simulink model "SSSTSMCC_SIM2augr"  (R2021a)
settings: Solver=ode23  StartTime=0.0  StopTime=T_s  RelTol=1e-3
InitFcn:
  | run('constant_velocity_trajectories_variable_angle_2.m')
StopFcn:
  | run('plot_response.m')
model workspace (MAT data in the model file):
  k1 = 828667.592561
  k10 = 1999999.9998
  k11 = 791466.214164
  k12 = 2711501.85139
  k13 = 1562664.14527
  k14 = 102615.336665
  k15 = 1.17580409761
  k16 = 0.102193267865
  k17 = 0.100015753782
  k18 = 0.0120332154736
  k19 = 1832731.57633
  k2 = 1.08080322166
  k20 = 1.1758040372
  k21 = 2464380.03061
  k22 = 64035.668317
  k23 = 215865.22677
  k24 = 1095290.61706
  k25 = 541886.168446
  k26 = 559452.633806
  k27 = 2923623.34482
  k28 = 1084341.04841
  k29 = 1.17580411876
  k3 = 3764225.72668
  k30 = 2999998.9242
  k31 = 18813308.9219
  k32 = 4784741.6959
  k33 = 196150293.659
  k34 = 125216769.116
  k35 = 9999998.9242
  k36 = 1.1758041248
  k37 = 3829.91588596
  k38 = 9683845.59238
  k39 = 71773726.6405
  k4 = 1104772.90021
  k40 = 2754807.69871
  k41 = 9999998.9242
  k42 = 29999998.9242
  k43 = 1999999998.92
  k44 = 550769.069765
  k5 = 1.1758040372
  k6 = 2511814.27977
  k7 = 1481585.56366
  k8 = 356837.383564
  k9 = 2398409.33781
values from neighbouring files (symbols this model uses):
  a_x = x(1:end-1)    [constant_velocity_trajectories.m]    (also in constant_velocity_trajectories_variable_angle.m; constant_velocity_trajectories_variable_angle_2.m)
  a_y = y(1:end-1)    [constant_velocity_trajectories.m]    (also in constant_velocity_trajectories_variable_angle.m; constant_velocity_trajectories_variable_angle_2.m)
  a_z = z(1:end-1)    [constant_velocity_trajectories.m]    (also in constant_velocity_trajectories_variable_angle.m; constant_velocity_trajectories_variable_angle_2.m)
  b_x = x(2:end)    [constant_velocity_trajectories.m]    (also in constant_velocity_trajectories_variable_angle.m; constant_velocity_trajectories_variable_angle_2.m)
  b_y = y(2:end)    [constant_velocity_trajectories.m]    (also in constant_velocity_trajectories_variable_angle.m; constant_velocity_trajectories_variable_angle_2.m)
  b_z = z(2:end)    [constant_velocity_trajectories.m]    (also in constant_velocity_trajectories_variable_angle.m; constant_velocity_trajectories_variable_angle_2.m)
  T = 2 * max(T_r)    [constant_velocity_trajectories.m]    (also in constant_velocity_trajectories_variable_angle.m; constant_velocity_trajectories_variable_angle_2.m)
  T_s = sum(T)    [constant_velocity_trajectories.m]    (also in constant_velocity_trajectories_variable_angle.m; constant_velocity_trajectories_variable_angle_2.m)
undefined symbols (not defined in the file or in its folder): k
libraries: simulink x17, pid_lib x6, sharedtransform x1, uavutilslib x1
settings Model: Creator=yig  LastModifiedBy=Traveler
settings SolverCC: AlgebraicLoopSolver=TrustRegion
settings DebuggingCC: AlgebraicLoopMsg=none  ArtificialAlgebraicLoopMsg=none  MaxConsecutiveZCsMsg=none  UnconnectedInputMsg=none  UnconnectedOutputMsg=none  UnconnectedLineMsg=none  ModelReferenceExtraNoncontSigs=none  OperatingPointInterfaceChecksumMismatchMsg=none  SFMachineParentedDataDiag=warning  ArithmeticOperatorsInVariantConditions=warning
settings ModelReferenceCC: EnableRefExpFcnMdlSchedulingChecks=off
settings SFSimCC: CustomCodeUndefinedFunction=UseInterfaceOnly
settings RTWCC: Description=Generic Real-Time Target

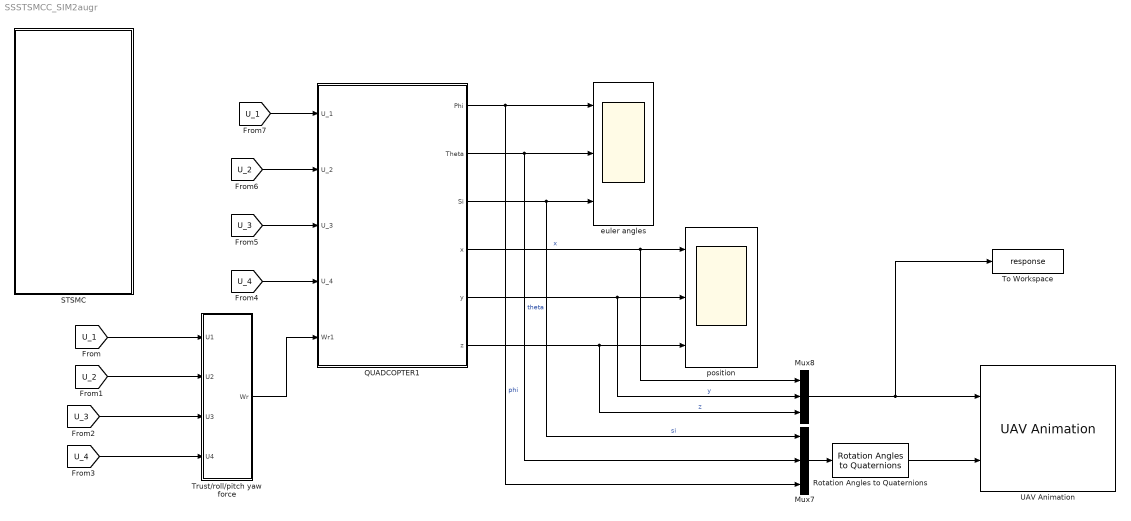
== system SSSTSMCC_SIM2augr ==
  Mux7 : Mux  Inputs=3
  Mux8 : Mux  Inputs=3
  QUADCOPTER1 : Subsystem
  Rotation Angles to Quaternions : sharedtransform/Rotation Angles to Quaternions  rotationOrder=ZYX  aMode=aMode
      settings: SourceProductBaseCode=AE,PW,DR,MT,UV,VE
  STSMC : Subsystem
  To Workspace : ToWorkspace  VariableName=response  SampleTime=-1
  Trust/roll/pitch yaw force : MATLAB Function  TreatAsAtomicUnit=on
  UAV Animation : uavutilslib/UAV Animation  UAVType=Multirotor  UAVSize=0.1  InertialZDirection=Up  SampleTime=0.1
      settings: SourceProductBaseCode=UV
  euler angles : Scope  NumInputPorts=3
  "position " : Scope  NumInputPorts=3
  wires:
  [U_1] -> QUADCOPTER1/1(U_1)
  [U_3] -> QUADCOPTER1/3(U_3)
  [U_2] -> QUADCOPTER1/2(U_2)
  [U_4] -> QUADCOPTER1/4(U_4)
  Trust/roll/pitch yaw force/1(Wr) -> QUADCOPTER1/5(Wr1)
  [U_1] -> Trust/roll/pitch yaw force/1(U1)
  [U_2] -> Trust/roll/pitch yaw force/2(U2)
  [U_3] -> Trust/roll/pitch yaw force/3(U3)
  [U_4] -> Trust/roll/pitch yaw force/4(U4)
  QUADCOPTER1/1(Phi) -> Mux7/3, euler angles/1  "phi"
  QUADCOPTER1/2(Theta) -> Mux7/2, euler angles/2  "theta"
  QUADCOPTER1/3(Si) -> Mux7/1, euler angles/3  "si"
  Mux8/1 -> To Workspace/1, UAV Animation/1
  Rotation Angles to Quaternions/1 -> UAV Animation/2
  QUADCOPTER1/6(z) -> "position "/3, Mux8/3  "z"
  QUADCOPTER1/5(y) -> "position "/2, Mux8/2  "y"
  QUADCOPTER1/4(x) -> Mux8/1, "position "/1  "x"
  Mux7/1 -> Rotation Angles to Quaternions/1

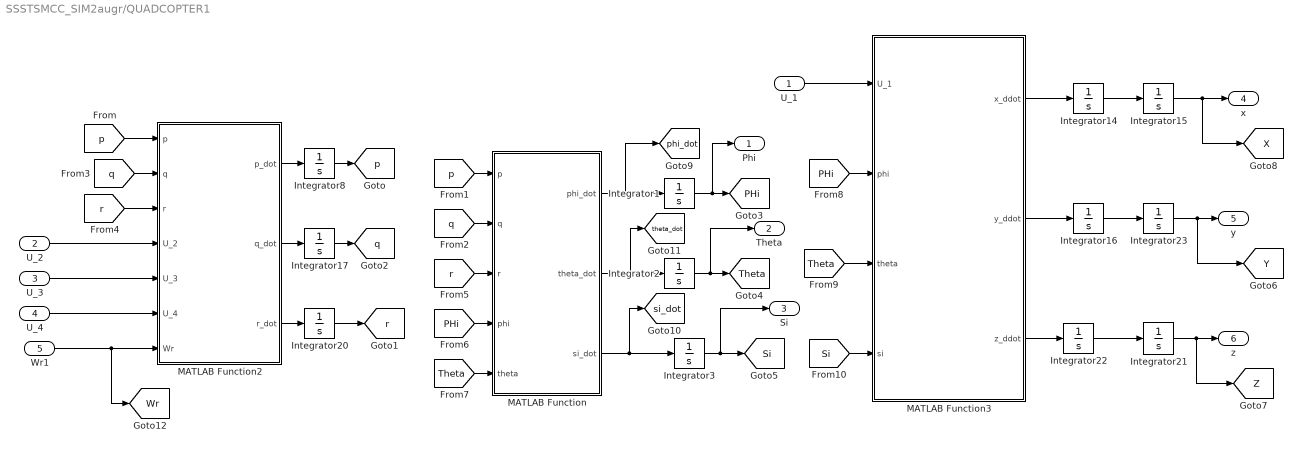
== system SSSTSMCC_SIM2augr/QUADCOPTER1 ==
  U_1 : Inport
  U_2 : Inport  Port=2
  U_3 : Inport  Port=3
  U_4 : Inport  Port=4
  Wr1 : Inport  Port=5
  Integrator1 : Integrator  WrapState=on  WrappedStateUpperValue=pi/3  WrappedStateLowerValue=-pi/3
  Integrator{14..16,22..23} (5 alike) : Integrator
  Integrator17 : Integrator  WrappedStateUpperValue=pi/3  WrappedStateLowerValue=-pi/3
  Integrator2 : Integrator  WrapState=on  WrappedStateUpperValue=pi/3  WrappedStateLowerValue=-pi/3
  Integrator20 : Integrator  WrappedStateUpperValue=pi/3  WrappedStateLowerValue=-pi/3
  Integrator21 : Integrator  UpperSaturationLimit=0
  Integrator3 : Integrator  WrapState=on
  Integrator8 : Integrator  WrappedStateUpperValue=pi/3  WrappedStateLowerValue=-pi/3
  MATLAB Function : MATLAB Function  TreatAsAtomicUnit=on
  MATLAB Function2 : MATLAB Function  TreatAsAtomicUnit=on
  MATLAB Function3 : MATLAB Function  TreatAsAtomicUnit=on
  Phi : Outport
  Theta : Outport  Port=2
  Si : Outport  Port=3
  x : Outport  Port=4
  y : Outport  Port=5
  z : Outport  Port=6
  tag scope: PHi=global, Si=global, Theta=global, Wr=global, X=global, Y=global, Z=global, p=global, phi_dot=global, q=global, r=global, si_dot=global, theta_dot=global
  wires:
  [p] -> MATLAB Function/1(p)
  [Si] -> MATLAB Function3/4(si)
  [Theta] -> MATLAB Function3/3(theta)
  Integrator2/1 -> Theta/1, [Theta]
  MATLAB Function/3(si_dot) -> [si_dot], Integrator3/1
  [r] -> MATLAB Function/3(r)
  [q] -> MATLAB Function/2(q)
  Integrator14/1 -> Integrator15/1
  Integrator3/1 -> Si/1, [Si]
  [q] -> MATLAB Function2/2(q)
  [r] -> MATLAB Function2/3(r)
  [Theta] -> MATLAB Function/5(theta)
  [p] -> MATLAB Function2/1(p)
  Integrator20/1 -> [r]
  Integrator8/1 -> [p]
  Integrator21/1 -> [Z], z/1
  MATLAB Function/1(phi_dot) -> [phi_dot], Integrator1/1
  Integrator1/1 -> Phi/1, [PHi]
  U_4/1 -> MATLAB Function2/6(U_4)
  [PHi] -> MATLAB Function3/2(phi)
  [PHi] -> MATLAB Function/4(phi)
  Integrator17/1 -> [q]
  Integrator22/1 -> Integrator21/1
  U_2/1 -> MATLAB Function2/4(U_2)
  Integrator15/1 -> [X], x/1
  MATLAB Function3/2(y_ddot) -> Integrator16/1
  MATLAB Function2/1(p_dot) -> Integrator8/1
  Integrator23/1 -> [Y], y/1
  Wr1/1 -> [Wr], MATLAB Function2/7(Wr)
  U_3/1 -> MATLAB Function2/5(U_3)
  MATLAB Function3/3(z_ddot) -> Integrator22/1
  MATLAB Function3/1(x_ddot) -> Integrator14/1
  MATLAB Function/2(theta_dot) -> [theta_dot], Integrator2/1
  MATLAB Function2/2(q_dot) -> Integrator17/1
  MATLAB Function2/3(r_dot) -> Integrator20/1
  U_1/1 -> MATLAB Function3/1(U_1)
  Integrator16/1 -> Integrator23/1

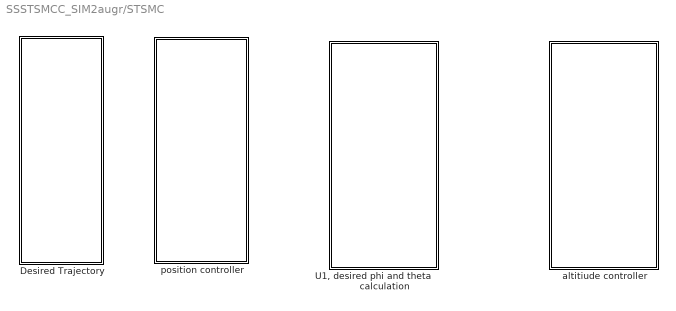
== system SSSTSMCC_SIM2augr/STSMC ==
  "             U1, desired phi and theta         calculation" : Subsystem
  " altitiude controller" : Subsystem  InitFcn="k = [3.1694    4.9704    4.6508    3.9758    2.6119    4.2532    1.3372    4.2753]"
  " position controller" : Subsystem
  Desired Trajectory : Subsystem

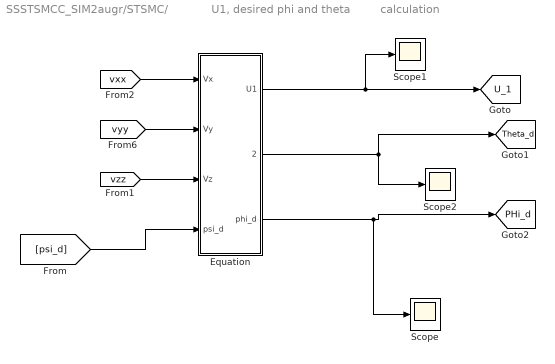
== system SSSTSMCC_SIM2augr/STSMC/             U1, desired phi and theta         calculation ==
  " Equation" : MATLAB Function  TreatAsAtomicUnit=on
  Scope : Scope
  Scope1 : Scope
  Scope2 : Scope
  tag scope: PHi_d=global, Theta_d=global, U_1=global
  wires:
  [vxx] -> " Equation"/1(Vx)
  [vyy] -> " Equation"/2(Vy)
  [vzz] -> " Equation"/3(Vz)
  [psi_d] -> " Equation"/4(psi_d)
  " Equation"/2(theta_d) -> [Theta_d], Scope2/1
  " Equation"/3(phi_d) -> Scope/1, [PHi_d]
  " Equation"/1(U1) -> Scope1/1, [U_1]

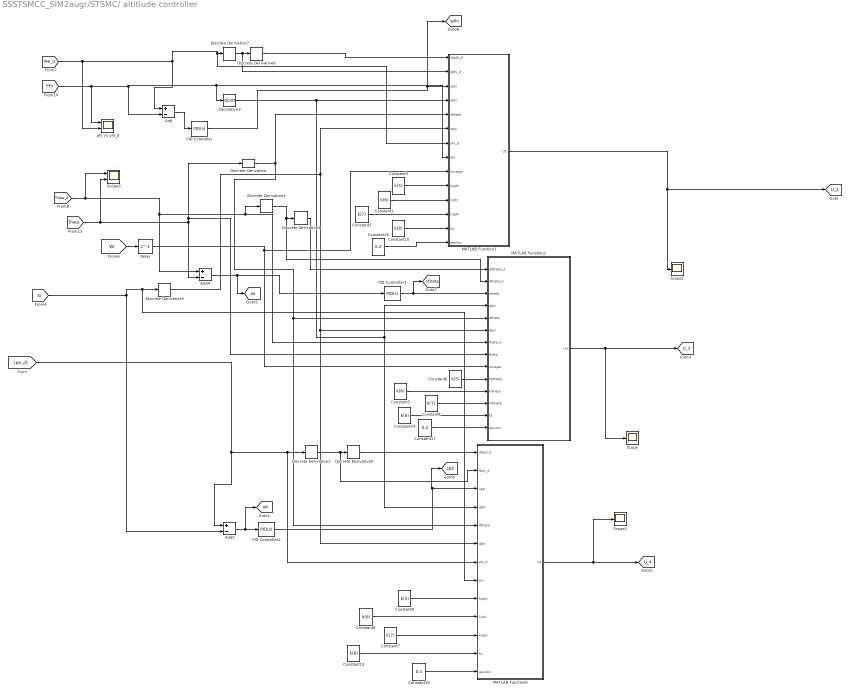
== system SSSTSMCC_SIM2augr/STSMC/ altitiude controller ==
  Add : Sum  Inputs=+-
  Add4 : Sum  Inputs=+-
  Add5 : Sum  Inputs=+-
  Constant1 : Constant  Value=k(6)  VectorParams1D=off
  Constant10 : Constant  Value=k(8)
  Constant13 : Constant  Value=k(8)
  Constant14 : Constant  Value=k(8)
  Constant17 : Constant  Value=0.2
  Constant19 : Constant  Value=0.1
  Constant2 : Constant  Value=k(7)
  Constant25 : Constant  Value=0.2
  Constant3 : Constant  Value=k(5)
  Constant4 : Constant  Value=k(7)
  Constant5 : Constant  Value=k(6)
  Constant6 : Constant  Value=k(5)
  Constant7 : Constant  Value=k(7)
  Constant8 : Constant  Value=k(6)
  Constant9 : Constant  Value=k(5)
  Delay : Delay  DelayLength=1  SampleTime=0.1
  Derivative3 : Derivative
  Discrete Derivative : simulink/Discrete/Discrete Derivative  gainval=0.1  ICPrevScaledInput=0.0  OutMin=[]  OutMax=[]  OutDataType=fixdt(1, 16)  OutScaling=2^-10  DoSatur=off
  Discrete Derivative{1..7} (7 alike) : simulink/Discrete/Discrete Derivative  gainval=1.0  ICPrevScaledInput=0.0  OutMin=[]  OutMax=[]  OutDataType=fixdt(1, 16)  OutScaling=2^-10  DoSatur=off
  MATLAB Function1 : MATLAB Function  TreatAsAtomicUnit=on
  MATLAB Function2 : MATLAB Function  TreatAsAtomicUnit=on
  MATLAB Function6 : MATLAB Function  TreatAsAtomicUnit=on
  PID Controller : pid_lib/PID Controller  Controller=PID  Form=Parallel  TimeDomain=Continuous-time  UseExternalTs=off  SampleTime=-1  IntegratorMethod=Forward Euler  FilterMethod=Forward Euler  ControllerParametersSource=internal  P=k(5)  I=k(6)  D=k(7)  UseFilter=on  N=100  TunerSelectOption=Transfer Function Based (PID Tuner App)  InitialConditionSource=internal  InitialConditionForIntegrator=0  InitialConditionForFilter=0  DifferentiatorICPrevScaledInput=0  ExternalReset=none  TrackingMode=off  Kt=1  LimitOutput=off  SatLimitsSource=internal  UpperSaturationLimit=inf  LowerSaturationLimit=-inf  LinearizeAsGain=on  AntiWindupMode=none  Kb=1  POutMin=[]  POutMax=[]  IOutMin=[]  IOutMax=[]  DOutMin=[]  DOutMax=[]  NOutMin=[]  NOutMax=[]  SumOutMin=[]  SumOutMax=[]  SaturationOutMin=[]  SaturationOutMax=[]  PParamMin=[]  PParamMax=[]  IParamMin=[]  IParamMax=[]  DParamMin=[]  DParamMax=[]  NParamMin=[]  NParamMax=[]  KbParamMin=[]  KbParamMax=[]  KtParamMin=[]  KtParamMax=[]  KbOutMin=[]  KbOutMax=[]  KtOutMin=[]  KtOutMax=[]  IntegratorOutMin=[]  IntegratorOutMax=[]  FilterOutMin=[]  FilterOutMax=[]  SumI1OutMin=[]  SumI1OutMax=[]  SumI2OutMin=[]  SumI2OutMax=[]  SumI3OutMin=[]  SumI3OutMax=[]  SumI4OutMin=[]  SumI4OutMax=[]  SumDOutMin=[]  SumDOutMax=[]  DifferentiatorOutMin=[]  DifferentiatorOutMax=[]  FilterDiffOutCoefMin=[]  FilterDiffOutCoefMax=[]  ReciprocalOutMin=[]  ReciprocalOutMax=[]  SumDenOutMin=[]  SumDenOutMax=[]  SumNumOutMin=[]  SumNumOutMax=[]  DivideOutMin=[]  DivideOutMax=[]  UdiffTsProdOutMin=[]  UdiffTsProdOutMax=[]  NTsProdOutMin=[]  NTsProdOutMax=[]  UintegralTsProdOutMin=[]  UintegralTsProdOutMax=[]  UngainTsProdOutMin=[]  UngainTsProdOutMax=[]  IntegratorContinuousStateAttributes=''  IntegratorStateMustResolveToSignalObject=off  IntegratorRTWStateStorageClass=Auto  FilterContinuousStateAttributes=''  FilterStateMustResolveToSignalObject=off  FilterRTWStateStorageClass=Auto  ParallelPVariant=InternalParameters  IdealPVariant=Disabled  IVariant=InternalParameters  DVariant=InternalParameters  IntegratorVariant=Continuous  SatVariant=Disabled  AWVariant=Passthrough  PCopyVariant=Disabled  TRVariant=Disabled  FdbkBlocksVariant=Forward  IdealPFdbkVariant=Disabled  SatFdbkVariant=Disabled  DerivativeFilterVariant=ContFilter  NVariant=InternalParameters  NCopyVariant=Disabled  FilterICVariant=InternalICsFilter  IntegratorICVariant=InternalICs  ExternalResetVariant=Disabled  TRSumVariant=Passthrough  SumFdbkVariant=Disabled  SumVariant=Sum_PID  TsampFilterVariant=InternalTs  TsampNgainVariant=Passthrough  TsampIntegralVariant=Passthrough  ExternalSaturationOutDataTypeStr=Inherit: Same as second input
  PID Controller1 : pid_lib/PID Controller  Controller=PID  Form=Parallel  TimeDomain=Continuous-time  UseExternalTs=off  SampleTime=-1  IntegratorMethod=Forward Euler  FilterMethod=Forward Euler  ControllerParametersSource=internal  P=k(5)  I=k(6)  D=k(7)  UseFilter=on  N=100  TunerSelectOption=Transfer Function Based (PID Tuner App)  InitialConditionSource=internal  InitialConditionForIntegrator=0  InitialConditionForFilter=0  DifferentiatorICPrevScaledInput=0  ExternalReset=none  TrackingMode=off  Kt=1  LimitOutput=off  SatLimitsSource=internal  UpperSaturationLimit=inf  LowerSaturationLimit=-inf  LinearizeAsGain=on  AntiWindupMode=none  Kb=1  POutMin=[]  POutMax=[]  IOutMin=[]  IOutMax=[]  DOutMin=[]  DOutMax=[]  NOutMin=[]  NOutMax=[]  SumOutMin=[]  SumOutMax=[]  SaturationOutMin=[]  SaturationOutMax=[]  PParamMin=[]  PParamMax=[]  IParamMin=[]  IParamMax=[]  DParamMin=[]  DParamMax=[]  NParamMin=[]  NParamMax=[]  KbParamMin=[]  KbParamMax=[]  KtParamMin=[]  KtParamMax=[]  KbOutMin=[]  KbOutMax=[]  KtOutMin=[]  KtOutMax=[]  IntegratorOutMin=[]  IntegratorOutMax=[]  FilterOutMin=[]  FilterOutMax=[]  SumI1OutMin=[]  SumI1OutMax=[]  SumI2OutMin=[]  SumI2OutMax=[]  SumI3OutMin=[]  SumI3OutMax=[]  SumI4OutMin=[]  SumI4OutMax=[]  SumDOutMin=[]  SumDOutMax=[]  DifferentiatorOutMin=[]  DifferentiatorOutMax=[]  FilterDiffOutCoefMin=[]  FilterDiffOutCoefMax=[]  ReciprocalOutMin=[]  ReciprocalOutMax=[]  SumDenOutMin=[]  SumDenOutMax=[]  SumNumOutMin=[]  SumNumOutMax=[]  DivideOutMin=[]  DivideOutMax=[]  UdiffTsProdOutMin=[]  UdiffTsProdOutMax=[]  NTsProdOutMin=[]  NTsProdOutMax=[]  UintegralTsProdOutMin=[]  UintegralTsProdOutMax=[]  UngainTsProdOutMin=[]  UngainTsProdOutMax=[]  IntegratorContinuousStateAttributes=''  IntegratorStateMustResolveToSignalObject=off  IntegratorRTWStateStorageClass=Auto  FilterContinuousStateAttributes=''  FilterStateMustResolveToSignalObject=off  FilterRTWStateStorageClass=Auto  ParallelPVariant=InternalParameters  IdealPVariant=Disabled  IVariant=InternalParameters  DVariant=InternalParameters  IntegratorVariant=Continuous  SatVariant=Disabled  AWVariant=Passthrough  PCopyVariant=Disabled  TRVariant=Disabled  FdbkBlocksVariant=Forward  IdealPFdbkVariant=Disabled  SatFdbkVariant=Disabled  DerivativeFilterVariant=ContFilter  NVariant=InternalParameters  NCopyVariant=Disabled  FilterICVariant=InternalICsFilter  IntegratorICVariant=InternalICs  ExternalResetVariant=Disabled  TRSumVariant=Passthrough  SumFdbkVariant=Disabled  SumVariant=Sum_PID  TsampFilterVariant=InternalTs  TsampNgainVariant=Passthrough  TsampIntegralVariant=Passthrough  ExternalSaturationOutDataTypeStr=Inherit: Same as second input
  PID Controller2 : pid_lib/PID Controller  Controller=PID  Form=Parallel  TimeDomain=Continuous-time  UseExternalTs=off  SampleTime=-1  IntegratorMethod=Forward Euler  FilterMethod=Forward Euler  ControllerParametersSource=internal  P=k(5)  I=k(6)  D=k(7)  UseFilter=on  N=100  TunerSelectOption=Transfer Function Based (PID Tuner App)  InitialConditionSource=internal  InitialConditionForIntegrator=0  InitialConditionForFilter=0  DifferentiatorICPrevScaledInput=0  ExternalReset=none  TrackingMode=off  Kt=1  LimitOutput=off  SatLimitsSource=internal  UpperSaturationLimit=inf  LowerSaturationLimit=-inf  LinearizeAsGain=on  AntiWindupMode=none  Kb=1  POutMin=[]  POutMax=[]  IOutMin=[]  IOutMax=[]  DOutMin=[]  DOutMax=[]  NOutMin=[]  NOutMax=[]  SumOutMin=[]  SumOutMax=[]  SaturationOutMin=[]  SaturationOutMax=[]  PParamMin=[]  PParamMax=[]  IParamMin=[]  IParamMax=[]  DParamMin=[]  DParamMax=[]  NParamMin=[]  NParamMax=[]  KbParamMin=[]  KbParamMax=[]  KtParamMin=[]  KtParamMax=[]  KbOutMin=[]  KbOutMax=[]  KtOutMin=[]  KtOutMax=[]  IntegratorOutMin=[]  IntegratorOutMax=[]  FilterOutMin=[]  FilterOutMax=[]  SumI1OutMin=[]  SumI1OutMax=[]  SumI2OutMin=[]  SumI2OutMax=[]  SumI3OutMin=[]  SumI3OutMax=[]  SumI4OutMin=[]  SumI4OutMax=[]  SumDOutMin=[]  SumDOutMax=[]  DifferentiatorOutMin=[]  DifferentiatorOutMax=[]  FilterDiffOutCoefMin=[]  FilterDiffOutCoefMax=[]  ReciprocalOutMin=[]  ReciprocalOutMax=[]  SumDenOutMin=[]  SumDenOutMax=[]  SumNumOutMin=[]  SumNumOutMax=[]  DivideOutMin=[]  DivideOutMax=[]  UdiffTsProdOutMin=[]  UdiffTsProdOutMax=[]  NTsProdOutMin=[]  NTsProdOutMax=[]  UintegralTsProdOutMin=[]  UintegralTsProdOutMax=[]  UngainTsProdOutMin=[]  UngainTsProdOutMax=[]  IntegratorContinuousStateAttributes=''  IntegratorStateMustResolveToSignalObject=off  IntegratorRTWStateStorageClass=Auto  FilterContinuousStateAttributes=''  FilterStateMustResolveToSignalObject=off  FilterRTWStateStorageClass=Auto  ParallelPVariant=InternalParameters  IdealPVariant=Disabled  IVariant=InternalParameters  DVariant=InternalParameters  IntegratorVariant=Continuous  SatVariant=Disabled  AWVariant=Passthrough  PCopyVariant=Disabled  TRVariant=Disabled  FdbkBlocksVariant=Forward  IdealPFdbkVariant=Disabled  SatFdbkVariant=Disabled  DerivativeFilterVariant=ContFilter  NVariant=InternalParameters  NCopyVariant=Disabled  FilterICVariant=InternalICsFilter  IntegratorICVariant=InternalICs  ExternalResetVariant=Disabled  TRSumVariant=Passthrough  SumFdbkVariant=Disabled  SumVariant=Sum_PID  TsampFilterVariant=InternalTs  TsampNgainVariant=Passthrough  TsampIntegralVariant=Passthrough  ExternalSaturationOutDataTypeStr=Inherit: Same as second input
  Scope : Scope
  Scope1 : Scope
  Scope2 : Scope
  Scope3 : Scope  NumInputPorts=2
  phi vs phi_d : Scope  NumInputPorts=2
  tag scope: U_2=global, U_3=global, U_4=global, e5=global, e6=global, sphi=global, spsi=global, stheta=global
  wires:
  [Theta] -> Scope3/2, Discrete Derivative/1, MATLAB Function2/8(theta), Add4/2
  [Wr] -> Delay/1
  [PHi_d] -> phi vs phi_d/2, Discrete Derivative7/1, MATLAB Function1/7(phi_d), Add/1
  [Si] -> MATLAB Function6/8(psi), Discrete Derivative5/1, Add5/2
  Discrete Derivative1/1 -> MATLAB Function6/2(dpsi_d), Discrete Derivative4/1
  Discrete Derivative/1 -> MATLAB Function1/5(dtheta), MATLAB Function6/5(dtheta), MATLAB Function2/5(dtheta)
  Derivative3/1 -> MATLAB Function6/4(dphi), MATLAB Function2/4(dphi), MATLAB Function1/4(dphi)
  [Theta_d] -> Scope3/1, Add4/1, MATLAB Function2/7(theta_d), Discrete Derivative3/1
  Discrete Derivative2/1 -> MATLAB Function2/1(ddtheta_d)
  Discrete Derivative3/1 -> Discrete Derivative2/1, MATLAB Function2/2(dtheta_d)
  Discrete Derivative4/1 -> MATLAB Function6/1(ddpsi_d)
  Discrete Derivative6/1 -> MATLAB Function1/1(ddphi_d)
  Discrete Derivative5/1 -> MATLAB Function2/6(dpsi), MATLAB Function6/6(dpsi), MATLAB Function1/6(dpsi)
  Discrete Derivative7/1 -> Discrete Derivative6/1, MATLAB Function1/2(dphi_d)
  [psi_d] -> Add5/1, MATLAB Function6/7(psi_d), Discrete Derivative1/1
  Constant10/1 -> MATLAB Function1/13(kp)
  Constant14/1 -> MATLAB Function2/13(kt)
  Constant13/1 -> MATLAB Function6/12(ks)
  [PHi] -> phi vs phi_d/1, Derivative3/1, MATLAB Function1/8(phi), Add/2
  PID Controller2/1 -> MATLAB Function6/3(spsi), [spsi]
  PID Controller/1 -> [sphi], MATLAB Function1/3(sphi)
  Constant25/1 -> MATLAB Function1/14(epsilon)
  Constant17/1 -> MATLAB Function2/14(epsilon)
  Constant19/1 -> MATLAB Function6/13(epsilon)
  Add/1 -> PID Controller/1
  Add4/1 -> [e5], PID Controller1/1
  Add5/1 -> [e6], PID Controller2/1
  Constant3/1 -> MATLAB Function1/10(kpphi)
  Constant1/1 -> MATLAB Function1/11(kiphi)
  Constant2/1 -> MATLAB Function1/12(kdphi)
  Constant6/1 -> MATLAB Function2/10(kptheta)
  Constant5/1 -> MATLAB Function2/11(kitheta)
  Constant4/1 -> MATLAB Function2/12(kdtheta)
  Constant9/1 -> MATLAB Function6/9(kppsi)
  Constant8/1 -> MATLAB Function6/10(kipsi)
  Constant7/1 -> MATLAB Function6/11(kdpsi)
  PID Controller1/1 -> MATLAB Function2/3(stheta), [stheta]
  MATLAB Function1/1(U2) -> [U_2], Scope1/1
  MATLAB Function2/1(U3) -> [U_3], Scope/1
  MATLAB Function6/1(U4) -> Scope2/1, [U_4]
  Delay/1 -> MATLAB Function2/9(omegar), MATLAB Function1/9(omegar)

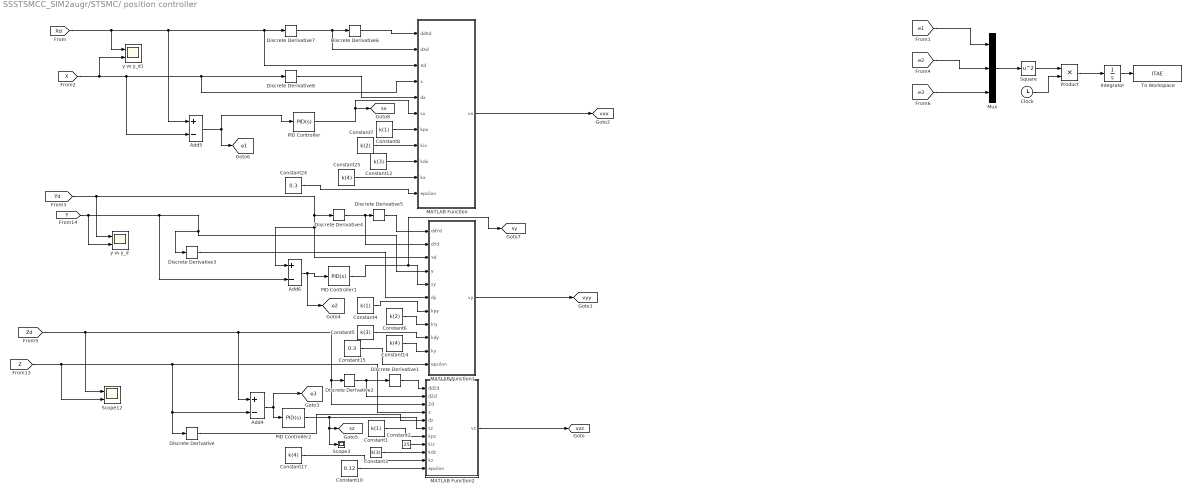
== system SSSTSMCC_SIM2augr/STSMC/ position controller ==
  Add4 : Sum  Inputs=+-
  Add5 : Sum  Inputs=+-
  Add6 : Sum  Inputs=+-
  Clock : Clock
  Constant1 : Constant  Value=k(1)
  Constant10 : Constant  Value=0.12
  Constant12 : Constant  Value=k(3)
  Constant14 : Constant  Value=k(4)
  Constant15 : Constant  Value=0.3
  Constant17 : Constant  Value=k(4)
  Constant2 : Constant  Value=25
  Constant24 : Constant  Value=0.3
  Constant25 : Constant  Value=k(4)
  Constant3 : Constant  Value=k(3)
  Constant4 : Constant  Value=k(1)
  Constant5 : Constant  Value=k(3)
  Constant6 : Constant  Value=k(2)
  Constant7 : Constant  Value=k(2)
  Constant8 : Constant  Value=k(1)
  Discrete Derivative{,1..8} (9 alike) : simulink/Discrete/Discrete Derivative  gainval=0.1  ICPrevScaledInput=0.0  OutMin=[]  OutMax=[]  OutDataType=fixdt(1, 16)  OutScaling=2^-10  DoSatur=off
  Integrator : Integrator
  MATLAB Function : MATLAB Function  TreatAsAtomicUnit=on
  MATLAB Function1 : MATLAB Function  TreatAsAtomicUnit=on
  MATLAB Function2 : MATLAB Function  TreatAsAtomicUnit=on
  Mux : Mux  Inputs=3
  PID Controller : pid_lib/PID Controller  Controller=PID  Form=Parallel  TimeDomain=Continuous-time  UseExternalTs=off  SampleTime=-1  IntegratorMethod=Forward Euler  FilterMethod=Forward Euler  ControllerParametersSource=internal  P=k(1)  I=k(2)  D=k(3)  UseFilter=on  N=100  TunerSelectOption=Transfer Function Based (PID Tuner App)  InitialConditionSource=internal  InitialConditionForIntegrator=0  InitialConditionForFilter=0  DifferentiatorICPrevScaledInput=0  ExternalReset=none  TrackingMode=off  Kt=1  LimitOutput=off  SatLimitsSource=internal  UpperSaturationLimit=inf  LowerSaturationLimit=-inf  LinearizeAsGain=on  AntiWindupMode=none  Kb=1  POutMin=[]  POutMax=[]  IOutMin=[]  IOutMax=[]  DOutMin=[]  DOutMax=[]  NOutMin=[]  NOutMax=[]  SumOutMin=[]  SumOutMax=[]  SaturationOutMin=[]  SaturationOutMax=[]  PParamMin=[]  PParamMax=[]  IParamMin=[]  IParamMax=[]  DParamMin=[]  DParamMax=[]  NParamMin=[]  NParamMax=[]  KbParamMin=[]  KbParamMax=[]  KtParamMin=[]  KtParamMax=[]  KbOutMin=[]  KbOutMax=[]  KtOutMin=[]  KtOutMax=[]  IntegratorOutMin=[]  IntegratorOutMax=[]  FilterOutMin=[]  FilterOutMax=[]  SumI1OutMin=[]  SumI1OutMax=[]  SumI2OutMin=[]  SumI2OutMax=[]  SumI3OutMin=[]  SumI3OutMax=[]  SumI4OutMin=[]  SumI4OutMax=[]  SumDOutMin=[]  SumDOutMax=[]  DifferentiatorOutMin=[]  DifferentiatorOutMax=[]  FilterDiffOutCoefMin=[]  FilterDiffOutCoefMax=[]  ReciprocalOutMin=[]  ReciprocalOutMax=[]  SumDenOutMin=[]  SumDenOutMax=[]  SumNumOutMin=[]  SumNumOutMax=[]  DivideOutMin=[]  DivideOutMax=[]  UdiffTsProdOutMin=[]  UdiffTsProdOutMax=[]  NTsProdOutMin=[]  NTsProdOutMax=[]  UintegralTsProdOutMin=[]  UintegralTsProdOutMax=[]  UngainTsProdOutMin=[]  UngainTsProdOutMax=[]  IntegratorContinuousStateAttributes=''  IntegratorStateMustResolveToSignalObject=off  IntegratorRTWStateStorageClass=Auto  FilterContinuousStateAttributes=''  FilterStateMustResolveToSignalObject=off  FilterRTWStateStorageClass=Auto  ParallelPVariant=InternalParameters  IdealPVariant=Disabled  IVariant=InternalParameters  DVariant=InternalParameters  IntegratorVariant=Continuous  SatVariant=Disabled  AWVariant=Passthrough  PCopyVariant=Disabled  TRVariant=Disabled  FdbkBlocksVariant=Forward  IdealPFdbkVariant=Disabled  SatFdbkVariant=Disabled  DerivativeFilterVariant=ContFilter  NVariant=InternalParameters  NCopyVariant=Disabled  FilterICVariant=InternalICsFilter  IntegratorICVariant=InternalICs  ExternalResetVariant=Disabled  TRSumVariant=Passthrough  SumFdbkVariant=Disabled  SumVariant=Sum_PID  TsampFilterVariant=InternalTs  TsampNgainVariant=Passthrough  TsampIntegralVariant=Passthrough  ExternalSaturationOutDataTypeStr=Inherit: Same as second input
  PID Controller1 : pid_lib/PID Controller  Controller=PID  Form=Parallel  TimeDomain=Continuous-time  UseExternalTs=off  SampleTime=-1  IntegratorMethod=Forward Euler  FilterMethod=Forward Euler  ControllerParametersSource=internal  P=k(1)  I=k(2)  D=k(3)  UseFilter=on  N=100  TunerSelectOption=Transfer Function Based (PID Tuner App)  InitialConditionSource=internal  InitialConditionForIntegrator=0  InitialConditionForFilter=0  DifferentiatorICPrevScaledInput=0  ExternalReset=none  TrackingMode=off  Kt=1  LimitOutput=off  SatLimitsSource=internal  UpperSaturationLimit=inf  LowerSaturationLimit=-inf  LinearizeAsGain=on  AntiWindupMode=none  Kb=1  POutMin=[]  POutMax=[]  IOutMin=[]  IOutMax=[]  DOutMin=[]  DOutMax=[]  NOutMin=[]  NOutMax=[]  SumOutMin=[]  SumOutMax=[]  SaturationOutMin=[]  SaturationOutMax=[]  PParamMin=[]  PParamMax=[]  IParamMin=[]  IParamMax=[]  DParamMin=[]  DParamMax=[]  NParamMin=[]  NParamMax=[]  KbParamMin=[]  KbParamMax=[]  KtParamMin=[]  KtParamMax=[]  KbOutMin=[]  KbOutMax=[]  KtOutMin=[]  KtOutMax=[]  IntegratorOutMin=[]  IntegratorOutMax=[]  FilterOutMin=[]  FilterOutMax=[]  SumI1OutMin=[]  SumI1OutMax=[]  SumI2OutMin=[]  SumI2OutMax=[]  SumI3OutMin=[]  SumI3OutMax=[]  SumI4OutMin=[]  SumI4OutMax=[]  SumDOutMin=[]  SumDOutMax=[]  DifferentiatorOutMin=[]  DifferentiatorOutMax=[]  FilterDiffOutCoefMin=[]  FilterDiffOutCoefMax=[]  ReciprocalOutMin=[]  ReciprocalOutMax=[]  SumDenOutMin=[]  SumDenOutMax=[]  SumNumOutMin=[]  SumNumOutMax=[]  DivideOutMin=[]  DivideOutMax=[]  UdiffTsProdOutMin=[]  UdiffTsProdOutMax=[]  NTsProdOutMin=[]  NTsProdOutMax=[]  UintegralTsProdOutMin=[]  UintegralTsProdOutMax=[]  UngainTsProdOutMin=[]  UngainTsProdOutMax=[]  IntegratorContinuousStateAttributes=''  IntegratorStateMustResolveToSignalObject=off  IntegratorRTWStateStorageClass=Auto  FilterContinuousStateAttributes=''  FilterStateMustResolveToSignalObject=off  FilterRTWStateStorageClass=Auto  ParallelPVariant=InternalParameters  IdealPVariant=Disabled  IVariant=InternalParameters  DVariant=InternalParameters  IntegratorVariant=Continuous  SatVariant=Disabled  AWVariant=Passthrough  PCopyVariant=Disabled  TRVariant=Disabled  FdbkBlocksVariant=Forward  IdealPFdbkVariant=Disabled  SatFdbkVariant=Disabled  DerivativeFilterVariant=ContFilter  NVariant=InternalParameters  NCopyVariant=Disabled  FilterICVariant=InternalICsFilter  IntegratorICVariant=InternalICs  ExternalResetVariant=Disabled  TRSumVariant=Passthrough  SumFdbkVariant=Disabled  SumVariant=Sum_PID  TsampFilterVariant=InternalTs  TsampNgainVariant=Passthrough  TsampIntegralVariant=Passthrough  ExternalSaturationOutDataTypeStr=Inherit: Same as second input
  PID Controller2 : pid_lib/PID Controller  Controller=PID  Form=Parallel  TimeDomain=Continuous-time  UseExternalTs=off  SampleTime=-1  IntegratorMethod=Forward Euler  FilterMethod=Forward Euler  ControllerParametersSource=internal  P=k(1)  I=k(2)  D=k(3)  UseFilter=on  N=100  TunerSelectOption=Transfer Function Based (PID Tuner App)  InitialConditionSource=internal  InitialConditionForIntegrator=0  InitialConditionForFilter=0  DifferentiatorICPrevScaledInput=0  ExternalReset=none  TrackingMode=off  Kt=1  LimitOutput=off  SatLimitsSource=internal  UpperSaturationLimit=inf  LowerSaturationLimit=-inf  LinearizeAsGain=on  AntiWindupMode=none  Kb=1  POutMin=[]  POutMax=[]  IOutMin=[]  IOutMax=[]  DOutMin=[]  DOutMax=[]  NOutMin=[]  NOutMax=[]  SumOutMin=[]  SumOutMax=[]  SaturationOutMin=[]  SaturationOutMax=[]  PParamMin=[]  PParamMax=[]  IParamMin=[]  IParamMax=[]  DParamMin=[]  DParamMax=[]  NParamMin=[]  NParamMax=[]  KbParamMin=[]  KbParamMax=[]  KtParamMin=[]  KtParamMax=[]  KbOutMin=[]  KbOutMax=[]  KtOutMin=[]  KtOutMax=[]  IntegratorOutMin=[]  IntegratorOutMax=[]  FilterOutMin=[]  FilterOutMax=[]  SumI1OutMin=[]  SumI1OutMax=[]  SumI2OutMin=[]  SumI2OutMax=[]  SumI3OutMin=[]  SumI3OutMax=[]  SumI4OutMin=[]  SumI4OutMax=[]  SumDOutMin=[]  SumDOutMax=[]  DifferentiatorOutMin=[]  DifferentiatorOutMax=[]  FilterDiffOutCoefMin=[]  FilterDiffOutCoefMax=[]  ReciprocalOutMin=[]  ReciprocalOutMax=[]  SumDenOutMin=[]  SumDenOutMax=[]  SumNumOutMin=[]  SumNumOutMax=[]  DivideOutMin=[]  DivideOutMax=[]  UdiffTsProdOutMin=[]  UdiffTsProdOutMax=[]  NTsProdOutMin=[]  NTsProdOutMax=[]  UintegralTsProdOutMin=[]  UintegralTsProdOutMax=[]  UngainTsProdOutMin=[]  UngainTsProdOutMax=[]  IntegratorContinuousStateAttributes=''  IntegratorStateMustResolveToSignalObject=off  IntegratorRTWStateStorageClass=Auto  FilterContinuousStateAttributes=''  FilterStateMustResolveToSignalObject=off  FilterRTWStateStorageClass=Auto  ParallelPVariant=InternalParameters  IdealPVariant=Disabled  IVariant=InternalParameters  DVariant=InternalParameters  IntegratorVariant=Continuous  SatVariant=Disabled  AWVariant=Passthrough  PCopyVariant=Disabled  TRVariant=Disabled  FdbkBlocksVariant=Forward  IdealPFdbkVariant=Disabled  SatFdbkVariant=Disabled  DerivativeFilterVariant=ContFilter  NVariant=InternalParameters  NCopyVariant=Disabled  FilterICVariant=InternalICsFilter  IntegratorICVariant=InternalICs  ExternalResetVariant=Disabled  TRSumVariant=Passthrough  SumFdbkVariant=Disabled  SumVariant=Sum_PID  TsampFilterVariant=InternalTs  TsampNgainVariant=Passthrough  TsampIntegralVariant=Passthrough  ExternalSaturationOutDataTypeStr=Inherit: Same as second input
  Product : Product
  Scope12 : Scope  NumInputPorts=2
  Scope3 : Scope
  Square : Math  Operator=square  SignedPower=on  SaturateOnIntegerOverflow=on
  To Workspace : ToWorkspace  VariableName=ITAE  SampleTime=-1
  y vs y_d : Scope  NumInputPorts=2
  y vs y_d1 : Scope  NumInputPorts=2
  tag scope: e1=global, e2=global, e3=global, sx=global, sy=global, sz=global, vxx=global, vyy=global, vzz=global
  wires:
  [Zd] -> Scope12/1, Discrete Derivative2/1, MATLAB Function2/3(Zd), Add4/1
  Discrete Derivative8/1 -> MATLAB Function/5(dx)
  Discrete Derivative3/1 -> MATLAB Function1/6(dy)
  [Z] -> Scope12/2, Discrete Derivative/1, Add4/2, MATLAB Function2/4(z)
  [Xd] -> y vs y_d1/1, Add5/1, Discrete Derivative7/1, MATLAB Function/3(Xd)
  Discrete Derivative/1 -> MATLAB Function2/5(dz)
  [X] -> y vs y_d1/2, Add5/2, MATLAB Function/4(x), Discrete Derivative8/1
  [Y] -> y vs y_d/2, Discrete Derivative3/1, MATLAB Function1/4(y), Add6/2
  Discrete Derivative1/1 -> MATLAB Function2/1(ddZd)
  Discrete Derivative5/1 -> MATLAB Function1/1(ddYd)
  Discrete Derivative7/1 -> Discrete Derivative6/1, MATLAB Function/2(dXd)
  Discrete Derivative6/1 -> MATLAB Function/1(ddXd)
  [Yd] -> y vs y_d/1, Discrete Derivative4/1, Add6/1, MATLAB Function1/3(Yd)
  Discrete Derivative2/1 -> Discrete Derivative1/1, MATLAB Function2/2(dZd)
  Discrete Derivative4/1 -> Discrete Derivative5/1, MATLAB Function1/2(dYd)
  PID Controller2/1 -> Scope3/1, [sz], MATLAB Function2/6(sz)
  Constant25/1 -> MATLAB Function/10(kx)
  Constant14/1 -> MATLAB Function1/10(ky)
  Constant17/1 -> MATLAB Function2/10(kz)
  PID Controller/1 -> MATLAB Function/6(sx), [sx]
  PID Controller1/1 -> [sy], MATLAB Function1/5(sy)
  Constant24/1 -> MATLAB Function/11(epsilon)
  Constant15/1 -> MATLAB Function1/11(epsilon)
  Constant10/1 -> MATLAB Function2/11(epsilon)
  Add5/1 -> PID Controller/1, [e1]
  Add6/1 -> [e2], PID Controller1/1
  Add4/1 -> PID Controller2/1, [e3]
  Constant1/1 -> MATLAB Function2/7(kpz)
  Constant2/1 -> MATLAB Function2/8(kiz)
  Constant4/1 -> MATLAB Function1/7(kpy)
  Constant6/1 -> MATLAB Function1/8(kiy)
  Constant5/1 -> MATLAB Function1/9(kdy)
  Constant8/1 -> MATLAB Function/7(kpx)
  Constant7/1 -> MATLAB Function/8(kix)
  Constant12/1 -> MATLAB Function/9(kdx)
  Constant3/1 -> MATLAB Function2/9(kdz)
  [e1] -> Mux/1
  [e2] -> Mux/2
  [e3] -> Mux/3
  Mux/1 -> Square/1
  Square/1 -> Product/1
  Clock/1 -> Product/2
  Product/1 -> Integrator/1
  Integrator/1 -> To Workspace/1
  MATLAB Function1/1(vy) -> [vyy]
  MATLAB Function/1(vx) -> [vxx]
  MATLAB Function2/1(vz) -> [vzz]

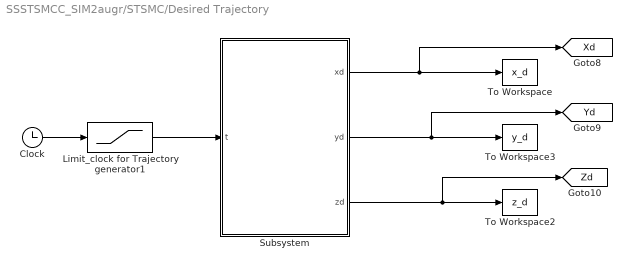
== system SSSTSMCC_SIM2augr/STSMC/Desired Trajectory ==
  Clock : Clock
  Limit_clock for Trajectory generator1 : Saturate  UpperLimit=T_s  LowerLimit=0
  Subsystem : Subsystem
  To Workspace : ToWorkspace  VariableName=x_d  SampleTime=0.1
  To Workspace2 : ToWorkspace  VariableName=z_d  SampleTime=0.1
  To Workspace3 : ToWorkspace  VariableName=y_d  SampleTime=0.1
  tag scope: Xd=global, Yd=global, Zd=global
  wires:
  Subsystem/2(yd) -> [Yd], To Workspace3/1
  Subsystem/3(zd) -> [Zd], To Workspace2/1
  Limit_clock for Trajectory generator1/1 -> Subsystem/1(t)
  Subsystem/1(xd) -> [Xd], To Workspace/1
  Clock/1 -> Limit_clock for Trajectory generator1/1

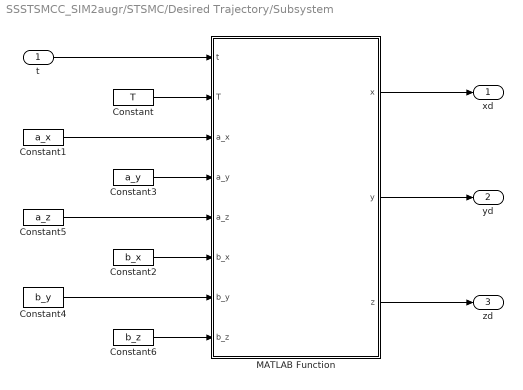
== system SSSTSMCC_SIM2augr/STSMC/Desired Trajectory/Subsystem ==
  t : Inport
  Constant : Constant  Value=T
  Constant1 : Constant  Value=a_x
  Constant2 : Constant  Value=b_x
  Constant3 : Constant  Value=a_y
  Constant4 : Constant  Value=b_y
  Constant5 : Constant  Value=a_z
  Constant6 : Constant  Value=b_z
  MATLAB Function : MATLAB Function  TreatAsAtomicUnit=on
  xd : Outport
  yd : Outport  Port=2
  zd : Outport  Port=3
  wires:
  Constant6/1 -> MATLAB Function/8(b_z)
  Constant4/1 -> MATLAB Function/7(b_y)
  MATLAB Function/3(z) -> zd/1
  Constant2/1 -> MATLAB Function/6(b_x)
  Constant/1 -> MATLAB Function/2(T)
  Constant3/1 -> MATLAB Function/4(a_y)
  Constant1/1 -> MATLAB Function/3(a_x)
  Constant5/1 -> MATLAB Function/5(a_z)
  MATLAB Function/2(y) -> yd/1
  MATLAB Function/1(x) -> xd/1
  t/1 -> MATLAB Function/1(t)

== matlab function SSSTSMCC_SIM2augr/QUADCOPTER1/MATLAB Function3 ==
  data: U_1 input; x_ddot output; phi input; theta input; si input; y_ddot output; z_ddot output
function[x_ddot,y_ddot,z_ddot] = fcn(U_1,phi,theta,si)
m=1;
g=9.81;
x_ddot=U_1*(cos(phi)*sin(theta)*cos(si) + sin(phi)*sin(si))/m;
y_ddot=U_1*(cos(phi)*sin(theta)*sin(si) - sin(phi)*cos(si))/m;
z_ddot=-g+U_1*(cos(phi)*cos(theta))/m;

== matlab function SSSTSMCC_SIM2augr/Trust//roll//pitch yaw force ==
  data: U1 input; U2 input; U3 input; U4 input; Wr output
function Wr  = fcn(U1,U2,U3,U4)
b=54.2*10^-6;
d=1.1*10^-6;
l=0.24;

Wr=-(sqrt((abs(0.25*(((U1/b)+((sqrt(2))*U2)/(b*l))+(((sqrt(2))*U3)/(b*l))+(U4/d))))))+sqrt((abs(0.25*(((U1/b)+((sqrt(2))*U2)/(b*l))-(((sqrt(2))*U3)/(b*l))-(U4/d)))))-(sqrt((abs(0.25*(((U1/b)-((sqrt(2))*U2)/(b*l))-(((sqrt(2))*U3)/(b*l))+(U4/d))))))+sqrt((abs(0.25*(((U1/b)-((sqrt(2))*U2)/(b*l))+(((sqrt(2))*U3)/(b*l))-(U4/d)))));

== matlab function SSSTSMCC_SIM2augr/STSMC/             U1, desired phi and theta         calculation/ Equation ==
  data: U1 output; Vx input; Vy input; Vz input; theta_d output; phi_d output; psi_d input

function [U1,theta_d,phi_d]  = fcn(Vx,Vy,Vz,psi_d)
m=1;%mass of the quadcopter
g=9.81;%gravitational acceleration
U1=m*sqrt(Vx^2+Vy^2+(Vz+g)^2);
theta_d=atan((cos(psi_d)*Vx+sin(psi_d)*Vy)/(Vz+g));
phi_d=atan(cos(theta_d)*(((sin(psi_d)*Vx-cos(psi_d)*Vy)/(Vz+g))));
end

== matlab function SSSTSMCC_SIM2augr/STSMC/Desired Trajectory/Subsystem/MATLAB Function ==
  data: t input; x output; T input; a_x input; a_y input; a_z input; b_x input; b_y input; y output; z output; b_z input
function [x, y, z] = design_trajectory(t, T, a_x, a_y, a_z, b_x, b_y, b_z)
    % Initialize output arrays
    x = zeros(size(t));
    y = zeros(size(t));
    z = zeros(size(t));
    
    % Loop through each time interval
    for i = 1:length(T)
        % Check if current time falls within the interval
        if (i == 1 && t <= T(i))
            [x, y, z] = helical_trajectory(t, a_x(i), a_y(i), a_z(i), b_z(i), T(i));
        elseif (i > 1 && t > sum(T(1:i-1)) && t <= sum(T(1:i)))
            [x, y, z] = constant_velocity_trajectory(t, sum(T(1:i-1)), sum(T(1:i)), a_x(i), a_y(i), a_z(i), b_x(i), b_y(i), b_z(i));
        end
    end
end

function [x, y, z] = helical_trajectory(t, a_x, a_y, a_z, b_z, T)
    % Define parameters for helical trajectory
    sd=0.5; rt=2;
    radius = rt + sd; % Example radius
    omega = 20* pi / T; % Angular velocity
    
    % Calculate the helical trajectory
    x = 0 + radius * cos(omega * t) ;
    y = 0 + radius * sin(omega * t) ;
    z = 0 + (b_z - a_z) * (t / T); % Helical movement in z
end

function [x, y, z] = constant_velocity_trajectory(t, T0, Tf, a_x, a_y, a_z, b_x, b_y, b_z)
    % Calculate the constant velocity trajectory
    duration = Tf - T0;
    
    % Calculate velocities
    vx = (b_x - a_x) / duration;
    vy = (b_y - a_y) / duration;
    vz = (b_z - a_z) / duration;
    
    % Calculate position at time t
    x = a_x + vx * (t - T0);
    y = a_y + vy * (t - T0);
    z = a_z + vz * (t - T0);
end

== matlab function SSSTSMCC_SIM2augr/STSMC/ position controller/MATLAB Function2 ==
  data: ddZd input; vz output; dZd input; Zd input; z input; dz input; sz input; kpz input; kiz input; kdz input; kz input; epsilon input



function vz = PIDSMCpositionz(ddZd,dZd,Zd,z,dz,sz,kpz,kiz,kdz,kz,epsilon)
% m=0.65;

vz= (1/kdz)*(kiz*(Zd-z)+kpz*(dZd-dz)+kdz*(ddZd))+kz*((sz)/(abs(sz)+epsilon));

== matlab function SSSTSMCC_SIM2augr/STSMC/ altitiude controller/MATLAB Function1 ==
  data: ddphi_d input; U2 output; dphi_d input; sphi input; dphi input; dtheta input; dpsi input; phi_d input; phi input; omegar input; kpphi input; kiphi input; kdphi input; kp input; epsilon input

function U2 = rollPIDSMC(ddphi_d,dphi_d,sphi,dphi,dtheta,dpsi,phi_d,phi,omegar,kpphi,kiphi,kdphi,kp,epsilon)

J=0.000104;
Ixx=0.0081;
Iyy=0.0081;
Izz=0.0142;
c1=((Iyy-Izz)/Ixx);
c3=((J)/Ixx);



U2 = (Ixx/kdphi)*(kiphi*(phi_d-phi)+kpphi*(dphi_d-dphi)+kdphi*(ddphi_d-c1*dtheta*dpsi+c3*dtheta*omegar))+kp*(sphi)/(abs(sphi)+epsilon);

== matlab function SSSTSMCC_SIM2augr/STSMC/ altitiude controller/MATLAB Function2 ==
  data: ddtheta_d input; dtheta_d input; U3 output; stheta input; dphi input; dtheta input; dpsi input; theta_d input; theta input; omegar input; kptheta input; kitheta input; kdtheta input; kt input; epsilon input

function U3 = pitchPIDSMC(ddtheta_d, dtheta_d, stheta, dphi, dtheta, dpsi, theta_d, theta, omegar, kptheta, kitheta, kdtheta,kt,epsilon)


Ixx=0.0081;
Iyy=0.0081;
Izz=0.0142;
J=0.000104;
c4=((Izz-Ixx)/Iyy);
c6=((J)/Iyy);

U3=(Iyy/kdtheta)*(kitheta*(theta_d-theta)+kptheta*(dtheta_d-dtheta)+kdtheta*(ddtheta_d-c4*dtheta*dpsi+c6*dphi*omegar))+kt*((stheta)/(abs(stheta)+epsilon));

== matlab function SSSTSMCC_SIM2augr/STSMC/ altitiude controller/MATLAB Function6 ==
  data: ddpsi_d input; U4 output; dpsi_d input; spsi input; dphi input; dtheta input; dpsi input; psi_d input; psi input; kppsi input; kipsi input; kdpsi input; ks input; epsilon input


function U4 = yawcontrol(ddpsi_d,dpsi_d,spsi,dphi,dtheta,dpsi,psi_d,psi,kppsi,kipsi,kdpsi,ks,epsilon)
Ixx=0.0081;
Iyy=0.0081;
Izz=0.0142;

c7=((Ixx-Iyy)/Izz);


U4 = (Izz/kdpsi)*(kipsi*(psi_d-psi)+kppsi*(dpsi_d-dpsi)+kdpsi*(ddpsi_d-c7*dphi*dtheta))+ks*((spsi)/(abs(spsi)+epsilon));

== matlab function SSSTSMCC_SIM2augr/STSMC/ position controller/MATLAB Function1 ==
  data: ddYd input; vy output; dYd input; Yd input; y input; sy input; dy input; kpy input; kiy input; kdy input; ky input; epsilon input

function vy = PIDSMCpositiony(ddYd,dYd,Yd,y,sy,dy,kpy,kiy,kdy,ky,epsilon)


% m=0.65;
vy= (1/kdy)*(kiy*(Yd-y)+kpy*(dYd-dy)+kdy*ddYd)+ky*((sy)/(abs(sy)+epsilon));

== matlab function SSSTSMCC_SIM2augr/STSMC/ position controller/MATLAB Function ==
  data: ddXd input; dXd input; vx output; Xd input; x input; dx input; sx input; kpx input; kix input; kdx input; kx input; epsilon input



function vx = PIDSMCpositionx(ddXd,dXd,Xd,x,dx,sx,kpx,kix,kdx,kx,epsilon)


% m=0;
vx= (1/kdx)*(kix*(Xd-x)+kpx*(dXd-dx)+kdx*(ddXd))+(kx*(sx)/(abs(sx)+epsilon));

== matlab function SSSTSMCC_SIM2augr/QUADCOPTER1/MATLAB Function ==
  data: p input; phi_dot output; q input; r input; phi input; theta input; theta_dot output; si_dot output
function [phi_dot,theta_dot,si_dot]= fcn(p,q,r,phi,theta)
phi_dot=p+q*sin(phi)*tan(theta)+r*cos(phi)*tan(theta);
theta_dot=q*cos(phi)-sin(phi)*r;
si_dot=q*sin(phi)*sec(theta)+r*cos(phi)*sec(theta);

== matlab function SSSTSMCC_SIM2augr/QUADCOPTER1/MATLAB Function2 ==
  data: p_dot output; q_dot output; r_dot output; p input; q input; r input; U_2 input; U_3 input; U_4 input; Wr input
function [p_dot,q_dot,r_dot]= fcn(p,q,r,U_2,U_3,U_4,Wr)
Ix=0.0081;
Iy=0.0081;
Iz=0.0142;
JTP=0.000104;
p_dot=((Iy-Iz)*q*r-(JTP*q*Wr))/Ix + U_2/Ix;
q_dot=((Iz-Ix)*p*r+U_3 +(JTP*p*Wr))/Iy;
r_dot=((Ix-Iy)*p*q)/Iz + U_4/Iz;
